simulink model "ut_traj_gen"  (R2021a)
settings: Solver=FixedStepDiscrete  StartTime=0.0  StopTime=600  RelTol=1e-3  EnableMultiTasking=on
undefined symbols (not defined in the file or in its folder): acc, DiscIntNeverNeededParam, feedrate, TotalNumBlock, Ts2
libraries: simulink x7
settings Model: Creator=Quoke  LastModifiedBy=chq
settings SolverCC: AutoInsertRateTranBlk=on
settings DataIOCC: SaveOutput=off  SaveTime=off
settings OptimizationCC: DefaultParameterBehavior=Inlined  InlineInvariantSignals=on  EnhancedBackFolding=on  PassReuseOutputArgsAs=Individual arguments  StateBitsets=on  DataBitsets=on  ZeroExternalMemoryAtStartup=off  ZeroInternalMemoryAtStartup=off  NoFixptDivByZeroProtection=on  LifeSpan=1  OptimizeBlockOrder=speed  DifferentSizesBufferReuse=on  EfficientTunableParamExpr=on
settings DebuggingCC: ParameterTunabilityLossMsg=error
settings HardwareCC: ProdBitPerPointer=32  ProdBitPerSizeT=32  ProdBitPerPtrDiffT=32  ProdLargestAtomicFloat=None  ProdIntDivRoundTo=Floor  ProdWordSize=32  ProdHWDeviceType=Generic->Custom
settings SFSimCC: MATLABDynamicMemAlloc=off
settings RTWCC: SystemTargetFile=ert.tlc  TLCOptions=-p0  GenCodeOnly=on  TemplateMakefile=ert_default_tmf  GenerateReport=on  RTWVerbose=off  IncludeHyperlinkInReport=on  LaunchReport=on
settings CodeAppCC: ForceParamTrailComments=on  IgnoreCustomStorageClasses=off  OperatorAnnotations=on  SimulinkDataObjDesc=on  SFDataObjDesc=on  CustomSymbolStrGlobalVar=rt$N$M  CustomSymbolStrType=$N$M  CustomSymbolStrFcn=$N$M$F  CustomSymbolStrMacro=$N$M  InsertBlockDesc=on
settings ERTTargetCC: TargetLangStandard=C99 (ISO)  CodeReplacementLibrary=ISO_C  GenerateSampleERTMain=on  IncludeMdlTerminateFcn=off  SuppressErrorStatus=on  SupportAbsoluteTime=off  PurelyIntegerCode=on  SupportNonFinite=off  SupportComplex=off  InlinedParameterPlacement=NonHierarchical  RootIOFormat=Structure reference  ERTCustomFileTemplate=example_file_process.tlc

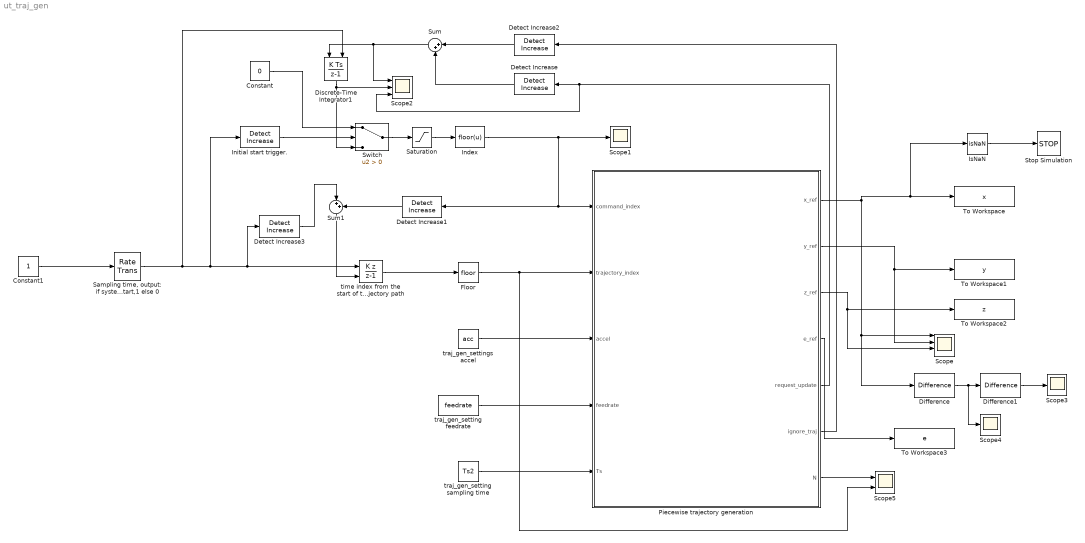
== system ut_traj_gen ==
  Constant : Constant  Value=0  SampleTime=Ts2
  Constant1 : Constant
  Detect Increase{,1..3} (4 alike) : simulink/Logic and Bit Operations/Detect Increase  vinit=0.0  OutDataTypeStr=boolean
  Difference : simulink/Discrete/Difference  ICPrevInput=0.0  OutMin=[]  OutMax=[]  OutDataType=fixdt(1, 16)  OutScaling=2^-10  DoSatur=off
  Difference1 : simulink/Discrete/Difference  ICPrevInput=0.0  OutMin=[]  OutMax=[]  OutDataType=fixdt(1, 16)  OutScaling=2^-10  DoSatur=off
  Discrete-Time Integrator1 : DiscreteIntegrator  gainval=1000  ExternalReset=rising  SampleTime=-1  OutDataTypeStr=uint32  ICPrevOutput=DiscIntNeverNeededParam  ICPrevScaledInput=DiscIntNeverNeededParam
  Floor : Rounding
  Index : Fcn  Expr=floor(u)
  Initial start trigger. : simulink/Logic and Bit Operations/Detect Increase  vinit=0.0  OutDataTypeStr=boolean
  IsNaN : RelationalOperator  Operator=isNaN  OutDataTypeStr=boolean  RndMeth=Simplest
  Piecewise trajectory generation : MATLAB Function  TreatAsAtomicUnit=on
  "Sampling time, output: if system start,1 else 0" : RateTransition  Integrity=off  Deterministic=off  OutPortSampleTime=Ts2
  Saturation : Saturate  UpperLimit=TotalNumBlock-1  LowerLimit=0
  Scope : Scope  NumInputPorts=4
  Scope1 : Scope
  Scope2 : Scope  NumInputPorts=3
  Scope3 : Scope
  Scope4 : Scope
  Scope5 : Scope  NumInputPorts=2
  Stop Simulation : Stop
  Sum : Sum  Inputs=|++
  Sum1 : Sum  Inputs=|++
  Switch : Switch  Criteria=u2 > Threshold
  To Workspace : ToWorkspace  VariableName=x  SaveFormat=Timeseries  SampleTime=-1
  To Workspace1 : ToWorkspace  VariableName=y  SaveFormat=Timeseries  SampleTime=-1
  To Workspace2 : ToWorkspace  VariableName=z  SaveFormat=Timeseries  SampleTime=-1
  To Workspace3 : ToWorkspace  VariableName=e  SaveFormat=Timeseries  SampleTime=-1
  time index from the start of trajectory path : DiscreteIntegrator  IntegratorMethod=Accumulation: Backward Euler  gainval=1  ExternalReset=rising  SampleTime=-1  ICPrevOutput=DiscIntNeverNeededParam  ICPrevScaledInput=DiscIntNeverNeededParam
  traj_gen_setting feedrate : Constant  Value=feedrate  SampleTime=Ts2
  traj_gen_setting sampling time : Constant  Value=Ts2  SampleTime=Ts2
  traj_gen_settings accel : Constant  Value=acc  SampleTime=Ts2
  wires:
  Piecewise trajectory generation/3(z_ref) -> Scope/3, To Workspace2/1
  Piecewise trajectory generation/2(y_ref) -> To Workspace1/1, Scope/2
  Piecewise trajectory generation/1(x_ref) -> IsNaN/1, To Workspace/1, Difference/1, Scope/1
  Difference/1 -> Scope4/1, Difference1/1
  Difference1/1 -> Scope3/1
  Floor/1 -> Scope5/2, Piecewise trajectory generation/2(trajectory_index)
  Detect Increase1/1 -> Sum1/2
  traj_gen_setting feedrate/1 -> Piecewise trajectory generation/4(feedrate)
  Initial start trigger./1 -> Switch/2
  Piecewise trajectory generation/5(request_update) -> Scope2/3, Detect Increase/1
  traj_gen_setting sampling time/1 -> Piecewise trajectory generation/5(Ts)
  traj_gen_settings accel/1 -> Piecewise trajectory generation/3(accel)
  Piecewise trajectory generation/6(ignore_traj) -> Detect Increase2/1
  Sum1/1 -> time index from the start of trajectory path/2
  Switch/1 -> Saturation/1
  Discrete-Time Integrator1/1 -> Switch/3, Scope2/2
  Constant/1 -> Switch/1
  time index from the start of trajectory path/1 -> Floor/1
  Saturation/1 -> Index/1
  Sum/1 -> Scope2/1, Discrete-Time Integrator1/1
  Index/1 -> Scope1/1, Piecewise trajectory generation/1(command_index), Detect Increase1/1
  Detect Increase/1 -> Sum/2
  "Sampling time, output: if system start,1 else 0"/1 -> Discrete-Time Integrator1/2, Detect Increase3/1, time index from the start of trajectory path/1, Initial start trigger./1
  Constant1/1 -> "Sampling time, output: if system start,1 else 0"/1
  Detect Increase2/1 -> Sum/1
  Piecewise trajectory generation/7(N) -> Scope5/1
  Detect Increase3/1 -> Sum1/1
  IsNaN/1 -> Stop Simulation/1
  Piecewise trajectory generation/4(e_ref) -> To Workspace3/1

== matlab function ut_traj_gen/Piecewise trajectory generation ==
  data: command_index input; x_ref output; trajectory_index input; accel input; feedrate input; y_ref output; z_ref output; e_ref output; request_update output; Ts input; simulink_commands parameter; ignore_traj output; N output
function [x_ref,y_ref,z_ref,e_ref,request_update,ignore_traj,N] = traj_generate(command_index,trajectory_index,accel,feedrate,Ts, simulink_commands)
    % Command is a compressed version of trajectory with trapz profile. 
    % it contains fs, fe and points. If feedrate, accel and Ts are the same
    % with that pre-generated, we could generate the identical trajectory.
    % [These parameters should be same with pre-trajectory generator! otherwise error may occurs] 
    % accel   [mm/s^2]  trajectory interpolate parameters, acceleration.
    % feedrate[mm/s]    trajectory interpolate parameters, feedrate.
    % Ts      [sec]     trajectory interpolate parameters, Ts.
    % [command struct]
    % points   [x;y;z;e] sets of gcode points contains 4 axes info.
    % fs       [mm/s]    trajectory start feedrate that has pre-calculated
    % fe       [mm/s]    trajectory end feedrate that has pre-calculated
    % length_N [num]     the number of points of interpolated trajectory
    % length_L [mm]      the trajectory piece length. (precisely evaluated by splineTBI)
    %
    % [Real time parameters]
    % trajectory_index  current index of generated trajectory piece
    % update_trajectory trajectory update request from last time stamp.
    % command_index     
    
    % Rebuild trajectory
    command = simulink_commands(command_index+1);
    command_points = command.points(command.points~=-114514);
    command_points = reshape(command_points,[4,length(command_points)/4]);
    traj_size = size(command_points);
    if(traj_size(2)==2)
        [current_pos,request_update,N] = linearTBI_rt(command_points(:,1),command_points(:,2),command.fs,command.fe,feedrate,accel,Ts,trajectory_index);
    else
        [current_pos,request_update,N] = splineTBI_rt(command_points,command.fs,command.fe,feedrate,accel,Ts,command.length_L,trajectory_index);
    end
    if(N==0)
        ignore_traj = 1;
    else
        ignore_traj = 0;
    end
    
    % Read xyze_ref based on current time.
    x_ref = current_pos(1);
    y_ref = current_pos(2);
    z_ref = current_pos(3);
    e_ref = current_pos(4);
    % Check if arrives at end. If so, push a request update request.
    if command_index == length(simulink_commands)
        request_update = false;
    end
end
